simulink model "oving3e"  (R2024b)
settings: Solver=ode2  StartTime=0.0  StopTime=3  FixedStep=.4  RelTol=1e-3
settings Model: Creator=tormod  LastModifiedBy=jorgen
settings DebuggingCC: UnconnectedInputMsg=warning  UnconnectedOutputMsg=warning  UnconnectedLineMsg=warning
settings ModelReferenceCC: EnableRefExpFcnMdlSchedulingChecks=on
settings RTWCC: GPUComputeCapability=3.5  DLArmComputeVersion=19.05

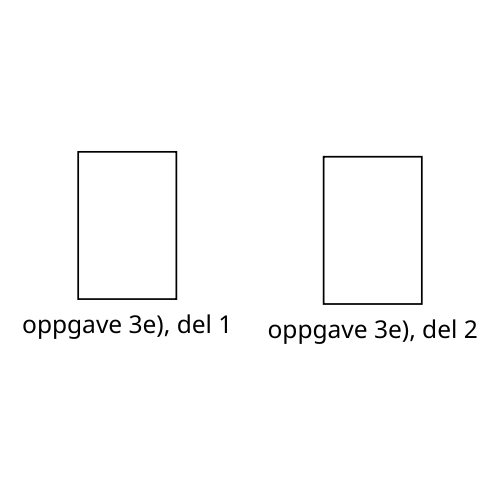
[thumbnail: Simulink's stored preview of the top-level diagram]
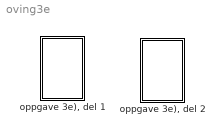
== system oving3e ==
  "oppgave 3e), del 1" : Subsystem
  "oppgave 3e), del 2" : Subsystem

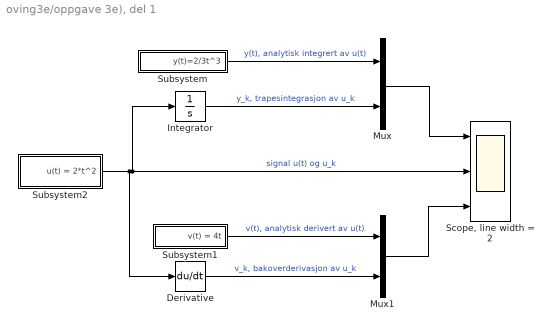
== system oving3e/oppgave 3e), del 1 ==
  Derivative : Derivative
  Integrator : Integrator
      settings: AttributesFormatString=IC = %<InitialCondition>
  Mux : Mux  Inputs=2
  Mux1 : Mux  Inputs=2
  "Scope, line width = 2" : Scope  NumInputPorts=3
  Subsystem : Subsystem
  Subsystem1 : Subsystem
  Subsystem2 : Subsystem
  wires:
  Integrator/1 -> Mux/2  "y_k, trapesintegrasjon av u_k"
  Derivative/1 -> Mux1/2  "v_k, bakoverderivasjon av u_k"
  Mux/1 -> "Scope, line width = 2"/1
  Mux1/1 -> "Scope, line width = 2"/3
  Subsystem/1(y(t)=2/3t^3) -> Mux/1  "y(t), analytisk integrert av u(t)"
  Subsystem1/1(v(t) = 4t) -> Mux1/1  "v(t), analytisk derivert av u(t)"
  Subsystem2/1(u(t) = 2*t^2) -> Derivative/1, "Scope, line width = 2"/2, Integrator/1  "signal u(t) og u_k"

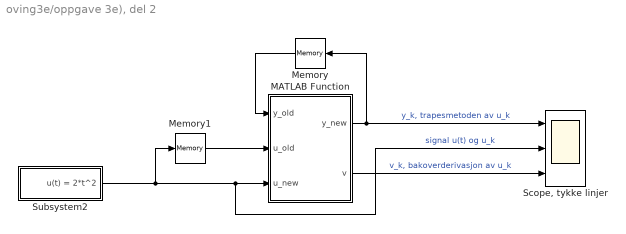
== system oving3e/oppgave 3e), del 2 ==
  MATLAB Function : MATLAB Function  TreatAsAtomicUnit=on
  Memory : Memory
      settings: AttributesFormatString=IC = %<InitialCondition>
  Memory1 : Memory
      settings: AttributesFormatString=IC = %<InitialCondition>
  "Scope, tykke linjer" : Scope  NumInputPorts=3
  Subsystem2 : Subsystem
  wires:
  MATLAB Function/1(y_new) -> Memory/1, "Scope, tykke linjer"/1  "y_k, trapesmetoden av u_k"
  MATLAB Function/2(v) -> "Scope, tykke linjer"/3  "v_k, bakoverderivasjon av u_k"
  Memory1/1 -> MATLAB Function/2(u_old)
  Memory/1 -> MATLAB Function/1(y_old)
  Subsystem2/1(u(t) = 2*t^2) -> Memory1/1, "Scope, tykke linjer"/2, MATLAB Function/3(u_new)  "signal u(t) og u_k"

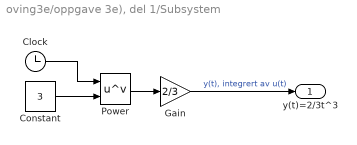
== system oving3e/oppgave 3e), del 1/Subsystem ==
  Clock : Clock
  Constant : Constant  Value=3
  Gain : Gain  Gain=2/3
  Power : Math  Operator=pow
  y(t)=2/3t^3 : Outport
  wires:
  Gain/1 -> y(t)=2/3t^3/1  "y(t), integrert av u(t)"
  Power/1 -> Gain/1
  Constant/1 -> Power/2
  Clock/1 -> Power/1

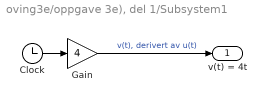
== system oving3e/oppgave 3e), del 1/Subsystem1 ==
  Clock : Clock
  Gain : Gain  Gain=4
  v(t) = 4t : Outport
  wires:
  Gain/1 -> v(t) = 4t/1  "v(t), derivert av u(t)"
  Clock/1 -> Gain/1

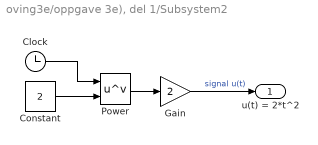
== system oving3e/oppgave 3e), del 1/Subsystem2 ==
  Clock : Clock
  Constant : Constant  Value=2
  Gain : Gain  Gain=2
  Power : Math  Operator=pow
  u(t) = 2*t^2 : Outport
  wires:
  Gain/1 -> u(t) = 2*t^2/1  "signal u(t)"
  Clock/1 -> Power/1
  Power/1 -> Gain/1
  Constant/1 -> Power/2

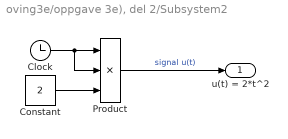
== system oving3e/oppgave 3e), del 2/Subsystem2 ==
  Clock : Clock
  Constant : Constant  Value=2
  Product : Product  Inputs=3
  u(t) = 2*t^2 : Outport
  wires:
  Product/1 -> u(t) = 2*t^2/1  "signal u(t)"
  Clock/1 -> Product/2, Product/1
  Constant/1 -> Product/3

== matlab function oving3e/oppgave 3e), del 2/MATLAB Function ==
  data: y_old input; u_old input; u_new input; y_new output; v output
function [y_new, v] = fcn(y_old,u_old,u_new)

% Tidssteg
Ts = 0.4;

% Trapesmetoden
y_new = y_old + Ts * 1/2 * (u_old + u_new);

% Bakoverderivasjon
v = (u_new - u_old)/Ts;

end
